simulink model "Simulacio_de_sistemas_continuos"  (R2017a)
settings: Solver=VariableStepAuto  StartTime=0.0  StopTime=10.0  RelTol=1e-3
settings Model: Creator=franj  LastModifiedBy=franj

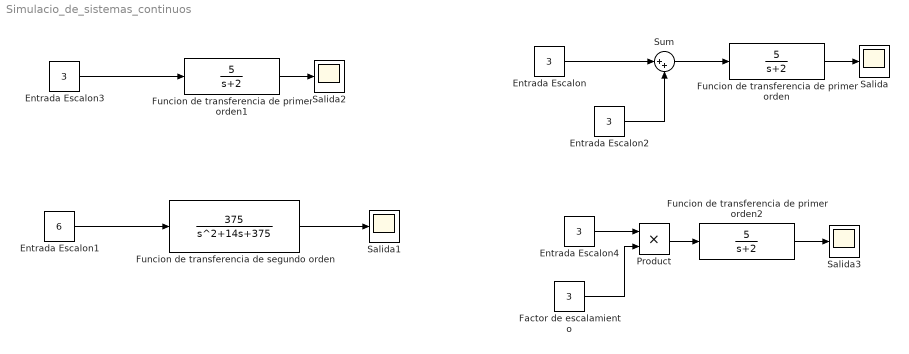
== system Simulacio_de_sistemas_continuos ==
  Entrada Escalon{,2..4} (4 alike) : Constant  Value=3
  Entrada Escalon1 : Constant  Value=6
  Factor de escalamiento : Constant  Value=3
  Funcion de transferencia de primer orden : TransferFcn  Numerator=[5]  Denominator=[1 2]
  Funcion de transferencia de primer orden1 : TransferFcn  Numerator=[5]  Denominator=[1 2]
  Funcion de transferencia de primer orden2 : TransferFcn  Numerator=[5]  Denominator=[1 2]
  Funcion de transferencia de segundo orden : TransferFcn  Numerator=[375]  Denominator=[1 14 375]
  Product : Product
  Salida{,1..3} (4 alike) : Scope
  Sum : Sum  Inputs=|++
  wires:
  Funcion de transferencia de primer orden/1 -> Salida/1
  Funcion de transferencia de segundo orden/1 -> Salida1/1
  Entrada Escalon1/1 -> Funcion de transferencia de segundo orden/1
  Entrada Escalon/1 -> Sum/1
  Sum/1 -> Funcion de transferencia de primer orden/1
  Entrada Escalon2/1 -> Sum/2
  Funcion de transferencia de primer orden1/1 -> Salida2/1
  Entrada Escalon3/1 -> Funcion de transferencia de primer orden1/1
  Funcion de transferencia de primer orden2/1 -> Salida3/1
  Product/1 -> Funcion de transferencia de primer orden2/1
  Entrada Escalon4/1 -> Product/1
  Factor de escalamiento/1 -> Product/2
